simulink model "path_gen"  (R2019b)
settings: Solver=VariableStepAuto  StartTime=0.0  StopTime=20  RelTol=1e-3
libraries: mobileRoboticsLib x3, dspsrcs4 x1, robotalgslib x1
settings Model: Creator=kpera  LastModifiedBy=kpera

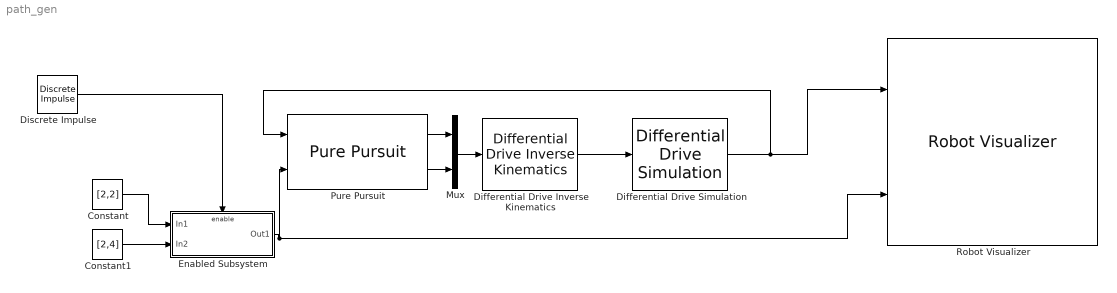
== system path_gen ==
  Constant : Constant  Value=[2,2]  VectorParams1D=off
  Constant1 : Constant  Value=[2,4]  VectorParams1D=off
  Differential Drive Inverse Kinematics : mobileRoboticsLib/Kinematic Models/Differential Drive/Differential Drive Inverse Kinematics  wheelRadius=0.1  wheelBase=0.5
      settings: SourceProductName=Mobile Robotics Simulation Toolbox
  Differential Drive Simulation : mobileRoboticsLib/Kinematic Models/Differential Drive/Differential Drive Simulation  wheelRadius=0.1  wheelBase=0.5  initX=2  initY=2  initAngle=90  Ts=0.05
      settings: SourceProductName=Mobile Robotics Simulation Toolbox
  Discrete Impulse : dspsrcs4/Discrete  Impulse  Delay=0  SampleTime=1  FrameSample=1  OutputFrames=off  dataType=double  isSigned=on  wordLen=16  udDataType=sfix(16)  fracBitsMode=Best precision  numFracBits=15  OutDataTypeStr=double  LastOutDataTypeStr=double
  Enabled Subsystem : Subsystem  TreatAsAtomicUnit=on
  Mux : Mux  Inputs=2
  Pure Pursuit : robotalgslib/Pure Pursuit  DesiredLinearVelocity=0.15  MaxAngularVelocity=0.1  LookaheadDistance=0.35  TargetDirPort=off  SimulateUsing=Code generation
      settings: SourceProductName=Navigation Toolbox  SourceProductBaseCode=NV
  Robot Visualizer : mobileRoboticsLib/Environments/Robot Visualizer  robotRadius=0  mapName=map  showTrajectory=on  hasWaypoints=on  hasLidar=off  sensorOffset=[ 0, 0 ]  scanAngles=[ -pi/4, 0, pi/4 ]  hasObjDetector=off  objDetectorOffset=[ 0, 0 ]  objDetectorAngle=0  objDetectorFOV=pi/4  objDetectorMaxRange=5  objectColors=[ 1, 0, 0; 0, 1, 0; 0, 0, 1 ]  objectMarkers='s'
  wires:
  Differential Drive Inverse Kinematics/1 -> Differential Drive Simulation/1
  Pure Pursuit/2 -> Mux/2
  Pure Pursuit/1 -> Mux/1
  Mux/1 -> Differential Drive Inverse Kinematics/1
  Differential Drive Simulation/1 -> Pure Pursuit/1, Robot Visualizer/1
  Enabled Subsystem/1(Out1) -> Pure Pursuit/2, Robot Visualizer/2
  Constant/1 -> Enabled Subsystem/1(In1)
  Constant1/1 -> Enabled Subsystem/2(In2)
  Discrete Impulse/1 -> Enabled Subsystem/Enable

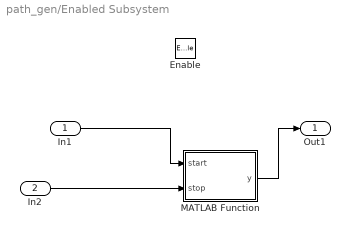
== system path_gen/Enabled Subsystem ==
  In1 : Inport
  In2 : Inport  Port=2
  Enable : EnablePort  PropagateVarSize=During execution
  MATLAB Function : MATLAB Function  TreatAsAtomicUnit=on
  Out1 : Outport
  wires:
  In1/1 -> MATLAB Function/1(start)
  MATLAB Function/1(y) -> Out1/1
  In2/1 -> MATLAB Function/2(stop)

== matlab function path_gen/Enabled Subsystem/MATLAB Function ==
  data: start input; y output size=[7,2] [..Inf]; stop input
function y = fcn(start, stop)
    path = [start,stop];
    flag = 1;
    while(flag == 1)
        s = load ('exampleMaps.mat');
        map = binaryOccupancyMap(s.simpleMap,2);
    %     R = 0.2;
    %     L = 0.1;
        map_inflate = copy(map);
        inflate(map_inflate,0.1)
        prm = mobileRobotPRM(map_inflate);
    %     prm.Map = map_inflate;
        prm.NumNodes = 50;
        prm.ConnectionDistance = 5;
        path = findpath(prm,start,stop);
        while isempty(path)
        % No feasible path found yet, increase the number of nodes
        prm.NumNodes = prm.NumNodes + 10;

        % Use the |update| function to re-create the PRM roadmap with the changed
        % attribute
        update(prm);

        % Search for a feasible path with the updated PRM
        path = findpath(prm, start, stop);
        end
        
        flag = 0;
    end
    y=path;
end
